simulink model "ECE371_Lab6_Simple"  (R2017a)
settings: Solver=ode3  StartTime=0.0  StopTime=Tf  FixedStep=0.01  RelTol=1e-3
libraries: simulink x1
settings Model: Creator=localmgr  LastModifiedBy=localmgr

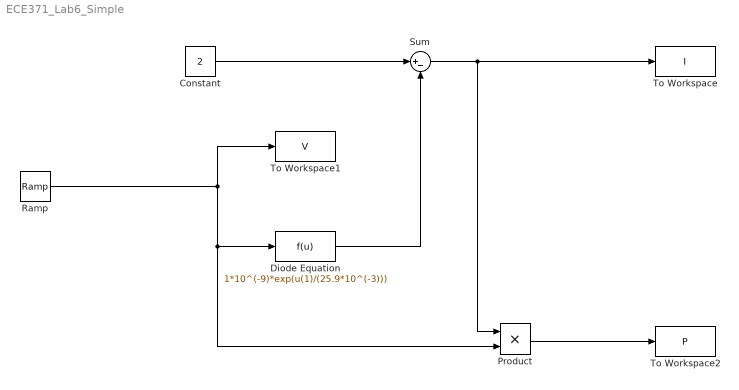
== system ECE371_Lab6_Simple ==
  Constant : Constant  Value=2
  "Diode Equation " : Fcn  Expr=1*10^(-9)*exp(u(1)/(25.9*10^(-3)))
  Product : Product
  Ramp : simulink/Sources/Ramp  slope=1  start=0  X0=0
  Sum : Sum  Inputs=|+-
  To Workspace : ToWorkspace  VariableName=I  SampleTime=-1
  To Workspace1 : ToWorkspace  VariableName=V  SampleTime=-1
  To Workspace2 : ToWorkspace  VariableName=P  SampleTime=-1
  wires:
  Constant/1 -> Sum/1
  Sum/1 -> To Workspace/1, Product/1
  Ramp/1 -> "Diode Equation "/1, Product/2, To Workspace1/1
  "Diode Equation "/1 -> Sum/2
  Product/1 -> To Workspace2/1
